simulink model "i_r303_med_1"  (Simulink 6.2)
settings: Solver=ode45  StartTime=0.0  StopTime=10  RelTol=1e-3
libraries: xbsIndex_r3 x540, xps_library x26, ddc_library x4, reorder_library x3, fft_library x2, pfb_library x2, simulink x1, adcscope_lib x1, delay_lib x1
(part 1 of 4)
settings Model: LastModifiedBy=dsp
settings DebuggingCC: SolverPrmCheckMsg=warning

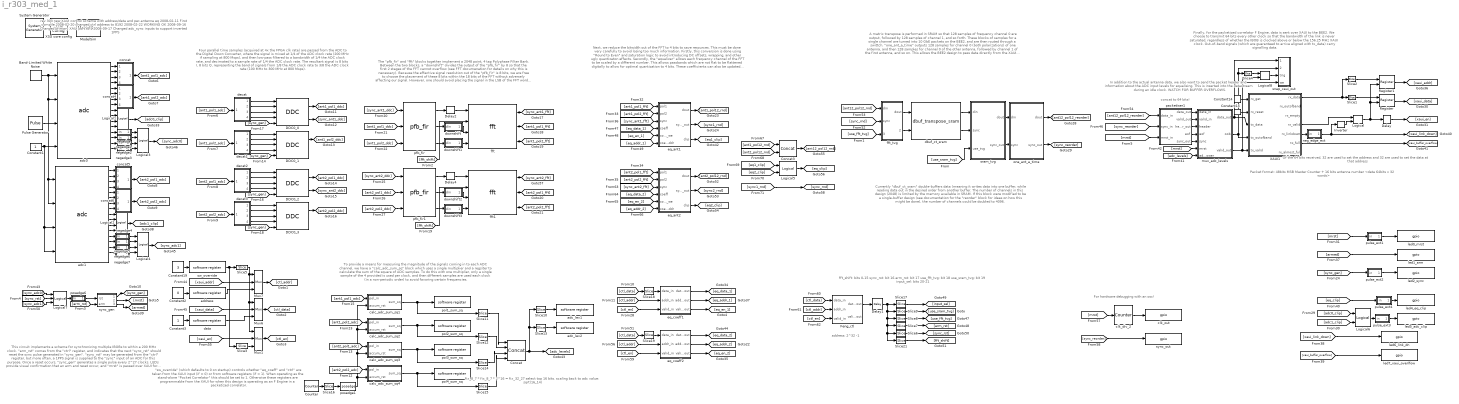
== system i_r303_med_1 ==
  note: rev 303
      | new XAUI control scheme with address/data
      | and per-antenna eq
      | 2008-02-11 First compile
      | 2008-02-20 changed ctrl address to 8192
      | 2008-02-22 WORKING OK
      | 2008-09-16 Changed primary XAUI port to 1
      | 2008-09-17 Changed adc_sync inputs to support inverted 1PPS
  note: This circuit implements a scheme for synchronizing
      | multiple IBOBs to within a 200 MHz clock.  "arm_rst"
      | comes from the "ctrl" register, and indicates that the
      | next "sync_rst" should reset the sync pulse generated
      | in "sync_gen".  "sync_rst" may be generated from
      | the "ctrl" register, but more often, a 1PPS signal is
      | supplied to the "sync" input of an ADC for this
      | purpose.  Once a reset occurs, "sync_gen" generates
      | a single pulse every 2^27 clocks.  LEDs provide visual
      | confirmation that an arm and reset occur, and "mrst"
      | is passed over XAUI for the purpose of informing
      | downstream logic in a packetized correlator that
      | a "master reset" has occurred.
  note: "sw_override" (which defaults to 0 on startup)
      | controls whether "eq_coeff" and "ctrl" are taken
      | from the XAUI input (if = 0) or from software
      | registers (if = 1).  When operating as the stand-alone
      | "Pocket Correlator" this should be set to 1.  Otherwise
      | these registers are programmable from the XAUI for
      | when this design is operating as  an F Engine
      | in a packetized correlator.
  note: Four parallel time samples (acquired at 4x the
      | FPGA clk rate) are passed from the ADC to the
      | Digital Down Converter, where the signal is mixed
      | at 1/4 of the ADC clock rate (200 MHz if sampling
      | at 800 Msps), and then low-pass filtered to a
      | bandwidth of 1/4 the ADC clock rate, and decimated
      | to a sample rate of 1/4 the ADC clock rate.  The
      | resultant signal is 8 bits I, 8 bits Q, representing the
      | band of signals from 1/8 the ADC clock rate to
      | 3/8 the ADC clock rate (100 MHz to 300 MHz at
      | 800 Msps).
  note: The "pfb_fir" and "fft" blocks together implement a 2048 point,
      | 4 tap Polyphase Filter Bank.  Between the two blocks, a "downshift"
      | divides the output of the "pfb_fir" by 8 so that the first 2 stages of
      | the FFT cannot overflow (see FFT documenation for details on why
      | this is necessary).  Because the effective signal resolution out of
      | the "pfb_fir" is 8 bits, we are free to choose the placement of
      | these 8 bits within the 18 bits of the FFT without adversely affecting
      | our signal.  However, one should avoid placing the signal in the LSB
      | of the FFT word because of rounding effects.  Thus, we downshift
      | only 3 bits.
  note: Next, we reduce the bitwidth out of the FFT to 4 bits to save resources.
      | This must be done very carefully to avoid losing too much information.
      | Firstly, this conversion is done using "Round to Even" and saturation
      | logic to avoid introducing DC offsets, wrapping, and other ugly quantizaton
      | effects.  Secondly, the "equalizer" allows each frequency channel of the
      | FFT to be scaled by a different number.  This allows passbands which are
      | not flat to be flattened digitally to allow for optimal quantization to 4 bits.
      | These coefficients can also be updated dynamically for gain control.
      | Coefficients can be dynamically written into the "equalizer" by
      | specifying the channel ("coeff_addr") and the value of the
      | coefficient ("coeff"), and then using "coeff_en" to write the
      | new coefficient into the equalization table.
  note: To provide a means for measuring the magnitude of the signals
      | coming in to each ADC channel, we have a "calc_adc_sum_sq"
      | block which uses a single multiplier and a regsiter to calculate
      | the sum of the square of ADC samples.  To do this with one
      | multiplier, only a single sample of the 4 provided is used
      | per clock, and then different samples are used each clock (in
      | a non-periodic order) to avoid favoring certain frequencies.
  note: A matrix transpose is performed in SRAM so that 128 samples of frequency
      | channel 0 are output, followed by 128 samples of channel 1, and so forth.
      | These blocks of samples for a single channel are turned into 10 GbE packets
      | on the BEE2, and are then routed through a swittch.  "one_ant_a_time"
      | outputs 128 samples for channel 0 (both polarizations) of one antenna,
      | and then 128 samples for channel 0 of the other antenna, followed by
      | channel 1 of the first antenna, and so on.  This allows the BEE2 design to
      | pass data directly from the XAUI into a packet containing 128 time samples
      | for 1 frequency from 1 antenna.
  note: Currently "dbuf_ct_sram" double-buffers data (meaning it writes data
      | into one buffer, while reading data out in the desired order from another
      | buffer.  The number of channels in this design (2048) is limited by the
      | memory available in SRAM.  If this block were modified to be a
      | single-buffer design (see documentation for the "reorder" block for
      | ideas on how this might be done), the number of channels could
      | be doubled to 4096.
  note: Finally, for the packetized correlator F Engine, data is sent over
      | XAUI to the BEE2.  We choose to transmit 64 bits every other clock
      | so that the bandwidth of the link is never saturated, regardless of whether
      | the IBOB is clocked above or below the 156.25 MHz XAUI clock.
      | Out-of-band signals (which are guaranteed to arrive aligned with
      | tx_data) carry signalling data.
  note: Of the 64 bits received, 32 are used to set the address
      | and 32 are used to set the data at that address
  note: fix_8_7 * fix_8_7 * 2^16 = fix_32_27
      | select top 16 bits.
      | scaling back to adc value: sqrt(16_14)
  note: In addition to the actual antenna data,
      | we also want to send the packet header
      | and information about the ADC input levels for equalising.
      | This is inserted into the datastream during an idle clock.
      | WATCH FOR BUFFER OVERFLOWS.
  note: Packet format:
      | 48bits MSB Master Counter + 16 bits antenna number
      | <data 64bits x 32 words>
  note: concat to 64 bits!
  note: fft_shift: bits 0-15
      | sync_rst: bit 16
      | arm_rst: bit 17
      | use_fft_tvg: bit 18
      | use_sram_tvg: bit 19
      | input_sel: bits 20-21
  note: For hardware debugging with an osc!
  note: address: 2^32 -1
  " System Generator" : xbsIndex_r3/ System Generator  Tag=genX  xilinxfamily=Virtex2P  part=xc2vp50  speed=-7  package=ff1152  synthesis_tool=XST  directory=./i_r303_med_1/sysgen  testbench=off  simulink_period=1  sysclk_period=5  incr_netlist=off  trim_vbits=Everywhere in SubSystem  dbl_ovrd=According to Block Masks  core_generation=According to Block Masks  run_coregen=off  deprecated_control=off  eval_field=0
      settings: AttributesFormatString=System\nGenerator
  Band-Limited White Noise : simulink/Sources/Band-Limited White Noise  Cov=[0.1]  Ts=0.1  seed=[23341]
  Concat : xbsIndex_r3/Concat  num_inputs=4  explicit_period=off  period=1  dbl_ovrd=off
  Concat3 : xbsIndex_r3/Concat  num_inputs=2  explicit_period=off  period=1  dbl_ovrd=off
  Constant1 : Constant
  Constant14 : xbsIndex_r3/Constant  const=1  equ=P=C  arith_type=Unsigned  n_bits=1  bin_pt=0  opselect=C  inp2=PCIN>>17  opr=+  inp1=P  carry=CIN  iostate=0  explicit_period=on  period=1  dbl_ovrd=off
  Constant15 : xbsIndex_r3/Constant  const=0  equ=P=C  arith_type=Unsigned  n_bits=1  bin_pt=0  opselect=C  inp2=PCIN>>17  opr=+  inp1=P  carry=CIN  iostate=0  explicit_period=on  period=1  dbl_ovrd=off
  Constant19 : Constant  Value=3
  Constant2 : Constant  Value=0
  Constant3 : Constant
  Counter : xbsIndex_r3/Counter  cnt_type=Free Running  n_bits=16  bin_pt=0  arith_type=Unsigned  start_count=0  cnt_to=Inf  cnt_by_val=1  operation=Up  explicit_period=off  period=1  load_pin=off  rst=off  en=off  dbl_ovrd=off  show_param=off  use_rpm=on  gen_core=off
      settings: xl_area=[0, 0, 0, 0, 0, 0, 0]
  DDC0_{0..3} (4 alike) : ddc_library/DDC  freq_div=4  lo_freq=1  num_inputs=4  lo_bitwidth=8  lpfir_coeff=".9 * [-0.0161   -0.0428   -0.0504   -0.0249    0.0354    0.1170    0.1948    0.2422    0.2422    0.1948    0.1170  0.0354   -0.0249   -0.0504   -0.0428   -0.0161]"  BitWidthOut=8  quantization="Round  (unbiased: Even Values)"  add_latency=1  mult_latency=2
  Delay : xbsIndex_r3/Delay  latency=1  reg_retiming=off  explicit_period=off  period=1  en=off  accept_only_valid=off  init_zero=on  dbl_ovrd=off  show_param=off
      settings: xl_area=[0, 0, 0, 0, 0, 0, 0]
  Delay1 : xbsIndex_r3/Delay  latency=1  reg_retiming=off  explicit_period=off  period=1  en=off  accept_only_valid=off  init_zero=on  dbl_ovrd=off  show_param=off
      settings: xl_area=[0, 0, 0, 0, 0, 0, 0]
  Delay2 : xbsIndex_r3/Delay  latency=2  reg_retiming=off  explicit_period=off  period=1  en=off  accept_only_valid=off  init_zero=on  dbl_ovrd=off  show_param=off
      settings: xl_area=[0, 0, 0, 0, 0, 0, 0]
  Delay4 : xbsIndex_r3/Delay  latency=2  reg_retiming=off  explicit_period=off  period=1  en=off  accept_only_valid=off  init_zero=on  dbl_ovrd=off  show_param=off
      settings: xl_area=[0, 0, 0, 0, 0, 0, 0]
  Feng_ctl : Subsystem  mask{addr_offset=8192}
      mask prompts: addr_offset "Address"
      mask init:
      | start_addr = (addr_offset);
      | fmtstr = sprintf('Mapped address: %d', start_addr);
      | set_param(gcb, 'AttributesFormatString', fmtstr);
      settings: AttributesFormatString=Mapped address: 8192
  Inverter : xbsIndex_r3/Inverter  latency=0  explicit_period=off  period=1  en=off  dbl_ovrd=off  show_param=off
      settings: xl_area=[0, 0, 0, 0, 0, 0, 0]
  Logical : xbsIndex_r3/Logical  logical_function=AND  inputs=2  precision=Full  arith_type=Unsigned  n_bits=8  bin_pt=2  align_bp=on  latency=0  explicit_period=off  period=1  en=off  dbl_ovrd=off  show_param=off
      settings: xl_area=[0, 0, 0, 0, 0, 0, 0]
  Logical{1..4} (4 alike) : xbsIndex_r3/Logical  logical_function=OR  inputs=4  precision=Full  arith_type=Unsigned  n_bits=8  bin_pt=2  align_bp=on  latency=1  explicit_period=off  period=1  en=off  dbl_ovrd=off  show_param=off
      settings: xl_area=[0, 0, 0, 0, 0, 0, 0]
  Logical5 : xbsIndex_r3/Logical  logical_function=OR  inputs=2  precision=Full  arith_type=Unsigned  n_bits=8  bin_pt=2  align_bp=on  latency=0  explicit_period=off  period=1  en=off  dbl_ovrd=off  show_param=off
      settings: xl_area=[0, 0, 0, 0, 0, 0, 0]
  Logical6 : xbsIndex_r3/Logical  logical_function=OR  inputs=2  precision=Full  arith_type=Unsigned  n_bits=8  bin_pt=2  align_bp=on  latency=1  explicit_period=off  period=1  en=off  dbl_ovrd=off  show_param=off
      settings: xl_area=[0, 0, 0, 0, 0, 0, 0]
  Logical7 : xbsIndex_r3/Logical  logical_function=OR  inputs=3  precision=Full  arith_type=Unsigned  n_bits=8  bin_pt=2  align_bp=on  latency=1  explicit_period=off  period=1  en=off  dbl_ovrd=off  show_param=off
      settings: xl_area=[0, 0, 0, 0, 0, 0, 0]
  Logical8 : xbsIndex_r3/Logical  logical_function=AND  inputs=2  precision=Full  arith_type=Unsigned  n_bits=8  bin_pt=2  align_bp=on  latency=0  explicit_period=off  period=1  en=off  dbl_ovrd=off  show_param=off
      settings: xl_area=[0, 0, 0, 0, 0, 0, 0]
  ModelSim : xbsIndex_r3/ModelSim  dir=./modelsim  waveform=on  leave_open=on  skip_compile=off  custom_scripts=off  startup_timeout=40
  Mux1 : xbsIndex_r3/Mux  inputs=2  precision=Full  arith_type="Signed  (2's comp)"  n_bits=8  bin_pt=2  quantization=Truncate  overflow=Wrap  latency=1  explicit_period=on  period=1  en=off  dbl_ovrd=off  show_param=off  mux_type=off  use_rpm=off  gen_core=off
      settings: xl_area=[0, 0, 0, 0, 0, 0, 0]
  Mux6 : xbsIndex_r3/Mux  inputs=2  precision=Full  arith_type="Signed  (2's comp)"  n_bits=8  bin_pt=2  quantization=Truncate  overflow=Wrap  latency=1  explicit_period=on  period=1  en=off  dbl_ovrd=off  show_param=off  mux_type=off  use_rpm=off  gen_core=off
      settings: xl_area=[0, 0, 0, 0, 0, 0, 0]
  Mux7 : xbsIndex_r3/Mux  inputs=2  precision=Full  arith_type="Signed  (2's comp)"  n_bits=8  bin_pt=2  quantization=Truncate  overflow=Wrap  latency=1  explicit_period=on  period=1  en=off  dbl_ovrd=off  show_param=off  mux_type=off  use_rpm=off  gen_core=off
      settings: xl_area=[0, 0, 0, 0, 0, 0, 0]
  Pulse Generator : DiscretePulseGenerator  Period=2^27
  Register : xbsIndex_r3/Register  init=0  reg_only_valid=off  explicit_period=off  period=1  rst=off  en=on  out_en=off  dbl_ovrd=off  show_param=off
      settings: xl_area=[0, 0, 0, 0, 0, 0, 0]
  Register1 : xbsIndex_r3/Register  init=0  reg_only_valid=off  explicit_period=off  period=1  rst=off  en=on  out_en=off  dbl_ovrd=off  show_param=off
      settings: xl_area=[0, 0, 0, 0, 0, 0, 0]
  Slice1 : xbsIndex_r3/Slice  mode=Lower Bit Location + Width  nbits=32  bit1=0  base1=MSB of Input  bit0=0  base0=LSB of Input  boolean_output=on  explicit_period=off  period=1  dbl_ovrd=off
  Slice10 : xbsIndex_r3/Slice  mode=Lower Bit Location + Width  nbits=32  bit1=0  base1=MSB of Input  bit0=0  base0=LSB of Input  boolean_output=off  explicit_period=off  period=1  dbl_ovrd=off
  Slice{11..12,14..15} (4 alike) : xbsIndex_r3/Slice  mode=Upper Bit Location + Width  nbits=16  bit1=0  base1=MSB of Input  bit0=0  base0=LSB of Input  boolean_output=off  explicit_period=off  period=1  dbl_ovrd=off
  Slice13 : xbsIndex_r3/Slice  mode=Lower Bit Location + Width  nbits=32  bit1=0  base1=MSB of Input  bit0=32  base0=LSB of Input  boolean_output=off  explicit_period=off  period=1  dbl_ovrd=off
  Slice16 : xbsIndex_r3/Slice  mode=Upper Bit Location + Width  nbits=1  bit1=0  base1=MSB of Input  bit0=19  base0=LSB of Input  boolean_output=on  explicit_period=off  period=1  dbl_ovrd=off
  Slice17 : xbsIndex_r3/Slice  mode=Lower Bit Location + Width  nbits=2  bit1=0  base1=MSB of Input  bit0=20  base0=LSB of Input  boolean_output=off  explicit_period=off  period=1  dbl_ovrd=off
  Slice18 : xbsIndex_r3/Slice  mode=Lower Bit Location + Width  nbits=17  bit1=0  base1=MSB of Input  bit0=0  base0=LSB of Input  boolean_output=off  explicit_period=off  period=1  dbl_ovrd=off
  Slice19 : xbsIndex_r3/Slice  mode=Lower Bit Location + Width  nbits=17  bit1=0  base1=MSB of Input  bit0=0  base0=LSB of Input  boolean_output=off  explicit_period=off  period=1  dbl_ovrd=off
  Slice2 : xbsIndex_r3/Slice  mode=Lower Bit Location + Width  nbits=32  bit1=0  base1=MSB of Input  bit0=32  base0=LSB of Input  boolean_output=off  explicit_period=off  period=1  dbl_ovrd=off
  Slice21 : xbsIndex_r3/Slice  mode=Lower Bit Location + Width  nbits=16  bit1=0  base1=MSB of Input  bit0=0  base0=LSB of Input  boolean_output=off  explicit_period=off  period=1  dbl_ovrd=off
  Slice3 : xbsIndex_r3/Slice  mode=Lower Bit Location + Width  nbits=1  bit1=0  base1=MSB of Input  bit0=1  base0=LSB of Input  boolean_output=on  explicit_period=off  period=1  dbl_ovrd=off
  Slice4 : xbsIndex_r3/Slice  mode=Lower Bit Location + Width  nbits=1  bit1=0  base1=MSB of Input  bit0=1  base0=LSB of Input  boolean_output=on  explicit_period=off  period=1  dbl_ovrd=off
  Slice5 : xbsIndex_r3/Slice  mode=Lower Bit Location + Width  nbits=1  bit1=0  base1=MSB of Input  bit0=0  base0=LSB of Input  boolean_output=off  explicit_period=off  period=1  dbl_ovrd=off
  Slice6 : xbsIndex_r3/Slice  mode=Lower Bit Location + Width  nbits=1  bit1=0  base1=MSB of Input  bit0=16  base0=LSB of Input  boolean_output=on  explicit_period=off  period=1  dbl_ovrd=off
  Slice7 : xbsIndex_r3/Slice  mode=Lower Bit Location + Width  nbits=1  bit1=0  base1=MSB of Input  bit0=17  base0=LSB of Input  boolean_output=on  explicit_period=off  period=1  dbl_ovrd=off
  Slice8 : xbsIndex_r3/Slice  mode=Lower Bit Location + Width  nbits=1  bit1=0  base1=MSB of Input  bit0=18  base0=LSB of Input  boolean_output=off  explicit_period=off  period=1  dbl_ovrd=off
  Slice9 : xbsIndex_r3/Slice  mode=Lower Bit Location + Width  nbits=1  bit1=0  base1=MSB of Input  bit0=19  base0=LSB of Input  boolean_output=off  explicit_period=off  period=1  dbl_ovrd=off
  XAUI1 : Subsystem  Tag=xps:xaui  AncestorBlock=xps_library/XAUI  mask{demux=1, port=iBOB:1, show_param=off, pre_emph=3, swing=800}
      mask prompts: show_param "---------------------- Show Implementation Parameters -----------------------------------------------------------------------------------"; pre_emph "Pre-emphasis"; swing "Differential swing"
      mask init:
      | xaui_mask;
      mask StyleString: popup(1|2),popup(iBOB:0|iBOB:1|BEE2_ctrl:0|BEE2_ctrl:1|BEE2_usr:0|BEE2_usr:1|BEE2_usr:2|BEE2_usr:3|CORR:0),checkbox,popup(0|1|2|3),popup(400|500|600|700|800)
      mask CallbackString:
      | ||myname=gcb;
      | if strcmp(get_param(myname, 'show_param'), 'on')
      |     set_param(myname, 'MaskVisibilities', {'on','on','on','on','on'});
      | else
      |     set_param(myname, 'MaskVisibilities', {'on','on','on','off','off'});
      | end||
  XSG core config : xps_library/XSG core config  Tag=xps:xsg  hw_sys=iBOB  ibob_linux=off  clk_src=adc0_clk  gpio_clk_io_group=iBOB:sma  gpio_clk_bit_index=0  clk_rate=200  sample_period=1  synthesis_tool=XST  mpc_type=powerpc405
  adc0 : xps_library/adc  Tag=xps:adc  adc_brd=iBOB:adc0  adc_clk_rate=600  adc_interleave=off  sample_period=1
  adc1 : xps_library/adc  Tag=xps:adc  adc_brd=iBOB:adc1  adc_clk_rate=600  adc_interleave=off  sample_period=1
  adc_lev1 : xps_library/software register  Tag=xps:sw_reg  io_dir=To Processor  arith_type=Unsigned  bitwidth=32  bin_pt=14  sample_period=1  gw_name=i_r303_med_1_adc_lev1_user_data_in
  adc_lev2 : xps_library/software register  Tag=xps:sw_reg  io_dir=To Processor  arith_type=Unsigned  bitwidth=32  bin_pt=14  sample_period=1  gw_name=i_r303_med_1_adc_lev2_user_data_in
  address : xps_library/software register  Tag=xps:sw_reg  io_dir=From Processor  arith_type=Unsigned  bitwidth=32  bin_pt=0  sample_period=1  gw_name=i_r303_med_1_address_user_data_out
  calc_adc_sum_sq1 : Subsystem
  calc_adc_sum_sq2 : Subsystem
  calc_adc_sum_sq3 : Subsystem
  calc_adc_sum_sq4 : Subsystem
  clk_div_2 : xbsIndex_r3/Counter  cnt_type=Free Running  n_bits=1  bin_pt=0  arith_type=Unsigned  start_count=0  cnt_to=Inf  cnt_by_val=1  operation=Up  explicit_period=off  period=1  load_pin=off  rst=on  en=off  dbl_ovrd=off  show_param=off  use_rpm=on  gen_core=off
      settings: xl_area=[0, 0, 0, 0, 0, 0, 0]
  clk_out : xps_library/gpio  Tag=xps:gpio  io_group=iBOB:sma  io_dir=out  arith_type=Unsigned  bitwidth=1  bin_pt=0  bit_index=0  sample_period=1  use_single_ended=off  use_ddr=off  reg_iob=on  reg_clk_phase=0  termination=None
  concat : Subsystem
  concat4 : Subsystem
  concat5 : Subsystem
  concat6 : Subsystem
  data : xps_library/software register  Tag=xps:sw_reg  io_dir=From Processor  arith_type=Unsigned  bitwidth=32  bin_pt=0  sample_period=1  gw_name=i_r303_med_1_data_user_data_out
  dbuf_ct_sram : reorder_library/dbuf_transpose_sram  length=2^11  numSpecs=128
      link override sync_delay/Constant: equ=P=C
      link override sync_delay/Constant1: equ=P=C
      link override sync_delay/Constant2: equ=P=C
      link override sync_delay/Constant3: equ=P=C
  decat : Subsystem
  decat1 : Subsystem
  decat2 : Subsystem
  decat3 : Subsystem
  downshift : Subsystem
  downshift1 : Subsystem
  downshift2 : Subsystem
  downshift3 : Subsystem
  eq_ant1 : Subsystem
  eq_ant2 : Subsystem
  eq_coeff1 : Subsystem  mask{addr_width=11, addr_offset=0}
      mask prompts: addr_width "Number of addresses (2^?)"; addr_offset "Address block offset (multiple of above)"
      mask init:
      | start_addr = 2^addr_width*(addr_offset);
      | end_addr = start_addr + 2^addr_width - 1;
      | fmtstr = sprintf('Mapped address range: %d-%d', start_addr,end_addr);
      | set_param(gcb, 'AttributesFormatString', fmtstr);
      settings: AttributesFormatString=Mapped address range: 0-2047
  eq_coeff2 : Subsystem  mask{addr_width=11, addr_offset=1}
      mask prompts: addr_width "Number of addresses (2^?)"; addr_offset "Address block offset (multiple of above)"
      mask init: same as i_r303_med_1/eq_coeff1
      settings: AttributesFormatString=Mapped address range: 2048-4095
  fft : fft_library/fft  FFTSize=11  BitWidth=18  n_inputs=0  quantization="Round  (unbiased: Even Values)"  overflow=Wrap  add_latency=1  mult_latency=2  bram_latency=2
  fft1 : fft_library/fft  FFTSize=11  BitWidth=18  n_inputs=0  quantization="Round  (unbiased: Even Values)"  overflow=Wrap  add_latency=1  mult_latency=2  bram_latency=2
  fft_tvg : Subsystem
  led0_mrst : xps_library/gpio  Tag=xps:gpio  io_group=iBOB:led  io_dir=out  arith_type=Boolean  bitwidth=1  bin_pt=0  bit_index=0  sample_period=1  use_single_ended=off  use_ddr=off  reg_iob=on  reg_clk_phase=0  termination=None
  led1_arm : xps_library/gpio  Tag=xps:gpio  io_group=iBOB:led  io_dir=out  arith_type=Boolean  bitwidth=1  bin_pt=0  bit_index=1  sample_period=1  use_single_ended=off  use_ddr=off  reg_iob=on  reg_clk_phase=0  termination=None
  led2_sync : xps_library/gpio  Tag=xps:gpio  io_group=iBOB:led  io_dir=out  arith_type=Boolean  bitwidth=1  bin_pt=0  bit_index=2  sample_period=1  use_single_ended=off  use_ddr=off  reg_iob=on  reg_clk_phase=0  termination=None
  led4_eq_clip : xps_library/gpio  Tag=xps:gpio  io_group=iBOB:led  io_dir=out  arith_type=Boolean  bitwidth=1  bin_pt=0  bit_index=4  sample_period=1  use_single_ended=off  use_ddr=off  reg_iob=on  reg_clk_phase=0  termination=None
  led5_adc_clip : xps_library/gpio  Tag=xps:gpio  io_group=iBOB:led  io_dir=out  arith_type=Boolean  bitwidth=1  bin_pt=0  bit_index=5  sample_period=1  use_single_ended=off  use_ddr=off  reg_iob=on  reg_clk_phase=0  termination=None
  led6_link_dn : xps_library/gpio  Tag=xps:gpio  io_group=iBOB:led  io_dir=out  arith_type=Unsigned  bitwidth=1  bin_pt=0  bit_index=6  sample_period=1  use_single_ended=off  use_ddr=off  reg_iob=on  reg_clk_phase=0  termination=None
  led7_xaui_overlfow : xps_library/gpio  Tag=xps:gpio  io_group=iBOB:led  io_dir=out  arith_type=Unsigned  bitwidth=1  bin_pt=0  bit_index=7  sample_period=1  use_single_ended=off  use_ddr=off  reg_iob=on  reg_clk_phase=0  termination=None
  mux_adc_levels : Subsystem  mask{wait_time=2000}
      mask prompts: wait_time "Attempt to insert antenna levels how many clocks after sync?"
  neg_edge_ext : Subsystem  mask{pulse_len=2^27}
      mask prompts: pulse_len "Length of Pulse"
      mask init:
      | bits = ceil(log2(pulse_len+1));
  negedge : Subsystem  Tag=Rising Edge Detector
  negedge1 : Subsystem  Tag=Rising Edge Detector
  negedge2 : Subsystem  Tag=Rising Edge Detector
  negedge3 : Subsystem  Tag=Rising Edge Detector
  negedge4 : Subsystem  Tag=Rising Edge Detector
  negedge5 : Subsystem  Tag=Rising Edge Detector
  negedge6 : Subsystem  Tag=Rising Edge Detector
  negedge7 : Subsystem  Tag=Rising Edge Detector
  one_ant_a_time : Subsystem
  packetiser1 : Subsystem  mask{nwrd_bits=5, ant_bits=1}
      mask prompts: nwrd_bits "Payload length: (in 64bit words) (2^n)"; ant_bits "Number of antennas on this link (2^n)"
      mask help: Package 32 bit data into 64 bits and identify data as coming from antenna 0 or 1
  pfb_fir : pfb_library/pfb_fir  PFBSize=11  TotalTaps=4  WindowType=hamming  n_inputs=0  MakeBiplex=on  BitWidthIn=8  BitWidthOut=18  CoeffBitWidth=8  CoeffDistMem=off  add_latency=1  mult_latency=2  bram_latency=2  quantization="Round  (unbiased: Even Values)"  fwidth=1
      link override pol1_in1_first_tap/sync_delay/Constant: equ=P=C
      link override pol1_in1_first_tap/sync_delay/Constant1: equ=P=C
      link override pol1_in1_first_tap/sync_delay/Constant2: equ=P=C
      link override pol1_in1_first_tap/sync_delay/Constant3: equ=P=C
      link override pol1_in1_tap10/sync_delay/Constant: equ=P=C
      link override pol1_in1_tap10/sync_delay/Constant1: equ=P=C
      link override pol1_in1_tap10/sync_delay/Constant2: equ=P=C
      link override pol1_in1_tap10/sync_delay/Constant3: equ=P=C
      link override pol1_in1_tap11/sync_delay/Constant: equ=P=C
      link override pol1_in1_tap11/sync_delay/Constant1: equ=P=C
      link override pol1_in1_tap11/sync_delay/Constant2: equ=P=C
      link override pol1_in1_tap11/sync_delay/Constant3: equ=P=C
      link override pol1_in1_tap12/sync_delay/Constant: equ=P=C
      link override pol1_in1_tap12/sync_delay/Constant1: equ=P=C
      link override pol1_in1_tap12/sync_delay/Constant2: equ=P=C
      link override pol1_in1_tap12/sync_delay/Constant3: equ=P=C
      link override pol1_in1_tap13/sync_delay/Constant: equ=P=C
      link override pol1_in1_tap13/sync_delay/Constant1: equ=P=C
      link override pol1_in1_tap13/sync_delay/Constant2: equ=P=C
      link override pol1_in1_tap13/sync_delay/Constant3: equ=P=C
      link override pol1_in1_tap14/sync_delay/Constant: equ=P=C
      link override pol1_in1_tap14/sync_delay/Constant1: equ=P=C
      link override pol1_in1_tap14/sync_delay/Constant2: equ=P=C
      link override pol1_in1_tap14/sync_delay/Constant3: equ=P=C
      link override pol1_in1_tap15/sync_delay/Constant: equ=P=C
      link override pol1_in1_tap15/sync_delay/Constant1: equ=P=C
      link override pol1_in1_tap15/sync_delay/Constant2: equ=P=C
      link override pol1_in1_tap15/sync_delay/Constant3: equ=P=C
      link override pol1_in1_tap2/sync_delay/Constant: equ=P=C
      link override pol1_in1_tap2/sync_delay/Constant1: equ=P=C
      link override pol1_in1_tap2/sync_delay/Constant2: equ=P=C
      link override pol1_in1_tap2/sync_delay/Constant3: equ=P=C
      link override pol1_in1_tap3/sync_delay/Constant: equ=P=C
      link override pol1_in1_tap3/sync_delay/Constant1: equ=P=C
      link override pol1_in1_tap3/sync_delay/Constant2: equ=P=C
      link override pol1_in1_tap3/sync_delay/Constant3: equ=P=C
      link override pol1_in1_tap4/sync_delay/Constant: equ=P=C
      link override pol1_in1_tap4/sync_delay/Constant1: equ=P=C
      link override pol1_in1_tap4/sync_delay/Constant2: equ=P=C
      link override pol1_in1_tap4/sync_delay/Constant3: equ=P=C
      link override pol1_in1_tap5/sync_delay/Constant: equ=P=C
      link override pol1_in1_tap5/sync_delay/Constant1: equ=P=C
      link override pol1_in1_tap5/sync_delay/Constant2: equ=P=C
      link override pol1_in1_tap5/sync_delay/Constant3: equ=P=C
      link override pol1_in1_tap6/sync_delay/Constant: equ=P=C
      link override pol1_in1_tap6/sync_delay/Constant1: equ=P=C
      link override pol1_in1_tap6/sync_delay/Constant2: equ=P=C
      link override pol1_in1_tap6/sync_delay/Constant3: equ=P=C
      link override pol1_in1_tap7/sync_delay/Constant: equ=P=C
      link override pol1_in1_tap7/sync_delay/Constant1: equ=P=C
      link override pol1_in1_tap7/sync_delay/Constant2: equ=P=C
      link override pol1_in1_tap7/sync_delay/Constant3: equ=P=C
      link override pol1_in1_tap8/sync_delay/Constant: equ=P=C
      link override pol1_in1_tap8/sync_delay/Constant1: equ=P=C
      link override pol1_in1_tap8/sync_delay/Constant2: equ=P=C
      link override pol1_in1_tap8/sync_delay/Constant3: equ=P=C
      link override pol1_in1_tap9/sync_delay/Constant: equ=P=C
      link override pol1_in1_tap9/sync_delay/Constant1: equ=P=C
      link override pol1_in1_tap9/sync_delay/Constant2: equ=P=C
      link override pol1_in1_tap9/sync_delay/Constant3: equ=P=C
      link override pol2_in1_first_tap/sync_delay/Constant: equ=P=C
      link override pol2_in1_first_tap/sync_delay/Constant1: equ=P=C
      link override pol2_in1_first_tap/sync_delay/Constant2: equ=P=C
      link override pol2_in1_first_tap/sync_delay/Constant3: equ=P=C
      link override pol2_in1_tap10/sync_delay/Constant: equ=P=C
      link override pol2_in1_tap10/sync_delay/Constant1: equ=P=C
      link override pol2_in1_tap10/sync_delay/Constant2: equ=P=C
      link override pol2_in1_tap10/sync_delay/Constant3: equ=P=C
      link override pol2_in1_tap11/sync_delay/Constant: equ=P=C
      link override pol2_in1_tap11/sync_delay/Constant1: equ=P=C
      link override pol2_in1_tap11/sync_delay/Constant2: equ=P=C
      link override pol2_in1_tap11/sync_delay/Constant3: equ=P=C
      link override pol2_in1_tap12/sync_delay/Constant: equ=P=C
      link override pol2_in1_tap12/sync_delay/Constant1: equ=P=C
      link override pol2_in1_tap12/sync_delay/Constant2: equ=P=C
      link override pol2_in1_tap12/sync_delay/Constant3: equ=P=C
      link override pol2_in1_tap13/sync_delay/Constant: equ=P=C
      link override pol2_in1_tap13/sync_delay/Constant1: equ=P=C
      link override pol2_in1_tap13/sync_delay/Constant2: equ=P=C
      link override pol2_in1_tap13/sync_delay/Constant3: equ=P=C
      link override pol2_in1_tap14/sync_delay/Constant: equ=P=C
      link override pol2_in1_tap14/sync_delay/Constant1: equ=P=C
      link override pol2_in1_tap14/sync_delay/Constant2: equ=P=C
      link override pol2_in1_tap14/sync_delay/Constant3: equ=P=C
      link override pol2_in1_tap15/sync_delay/Constant: equ=P=C
      link override pol2_in1_tap15/sync_delay/Constant1: equ=P=C
      link override pol2_in1_tap15/sync_delay/Constant2: equ=P=C
      link override pol2_in1_tap15/sync_delay/Constant3: equ=P=C
      link override pol2_in1_tap2/sync_delay/Constant: equ=P=C
      link override pol2_in1_tap2/sync_delay/Constant1: equ=P=C
      link override pol2_in1_tap2/sync_delay/Constant2: equ=P=C
      link override pol2_in1_tap2/sync_delay/Constant3: equ=P=C
      link override pol2_in1_tap3/sync_delay/Constant: equ=P=C
      link override pol2_in1_tap3/sync_delay/Constant1: equ=P=C
      link override pol2_in1_tap3/sync_delay/Constant2: equ=P=C
      link override pol2_in1_tap3/sync_delay/Constant3: equ=P=C
      link override pol2_in1_tap4/sync_delay/Constant: equ=P=C
      link override pol2_in1_tap4/sync_delay/Constant1: equ=P=C
      link override pol2_in1_tap4/sync_delay/Constant2: equ=P=C
      link override pol2_in1_tap4/sync_delay/Constant3: equ=P=C
      link override pol2_in1_tap5/sync_delay/Constant: equ=P=C
      link override pol2_in1_tap5/sync_delay/Constant1: equ=P=C
      link override pol2_in1_tap5/sync_delay/Constant2: equ=P=C
      link override pol2_in1_tap5/sync_delay/Constant3: equ=P=C
      link override pol2_in1_tap6/sync_delay/Constant: equ=P=C
      link override pol2_in1_tap6/sync_delay/Constant1: equ=P=C
      link override pol2_in1_tap6/sync_delay/Constant2: equ=P=C
      link override pol2_in1_tap6/sync_delay/Constant3: equ=P=C
      link override pol2_in1_tap7/sync_delay/Constant: equ=P=C
      link override pol2_in1_tap7/sync_delay/Constant1: equ=P=C
      link override pol2_in1_tap7/sync_delay/Constant2: equ=P=C
      link override pol2_in1_tap7/sync_delay/Constant3: equ=P=C
      link override pol2_in1_tap8/sync_delay/Constant: equ=P=C
      link override pol2_in1_tap8/sync_delay/Constant1: equ=P=C
      link override pol2_in1_tap8/sync_delay/Constant2: equ=P=C
      link override pol2_in1_tap8/sync_delay/Constant3: equ=P=C
      link override pol2_in1_tap9/sync_delay/Constant: equ=P=C
      link override pol2_in1_tap9/sync_delay/Constant1: equ=P=C
      link override pol2_in1_tap9/sync_delay/Constant2: equ=P=C
      link override pol2_in1_tap9/sync_delay/Constant3: equ=P=C
  pfb_fir1 : pfb_library/pfb_fir  PFBSize=11  TotalTaps=4  WindowType=hamming  n_inputs=0  MakeBiplex=on  BitWidthIn=8  BitWidthOut=18  CoeffBitWidth=8  CoeffDistMem=off  add_latency=1  mult_latency=2  bram_latency=2  quantization="Round  (unbiased: Even Values)"  fwidth=1
      link override pol1_in1_first_tap/sync_delay/Constant: equ=P=C
      link override pol1_in1_first_tap/sync_delay/Constant1: equ=P=C
      link override pol1_in1_first_tap/sync_delay/Constant2: equ=P=C
      link override pol1_in1_first_tap/sync_delay/Constant3: equ=P=C
      link override pol1_in1_tap10/sync_delay/Constant: equ=P=C
      link override pol1_in1_tap10/sync_delay/Constant1: equ=P=C
      link override pol1_in1_tap10/sync_delay/Constant2: equ=P=C
      link override pol1_in1_tap10/sync_delay/Constant3: equ=P=C
      link override pol1_in1_tap11/sync_delay/Constant: equ=P=C
      link override pol1_in1_tap11/sync_delay/Constant1: equ=P=C
      link override pol1_in1_tap11/sync_delay/Constant2: equ=P=C
      link override pol1_in1_tap11/sync_delay/Constant3: equ=P=C
      link override pol1_in1_tap12/sync_delay/Constant: equ=P=C
      link override pol1_in1_tap12/sync_delay/Constant1: equ=P=C
      link override pol1_in1_tap12/sync_delay/Constant2: equ=P=C
      link override pol1_in1_tap12/sync_delay/Constant3: equ=P=C
      link override pol1_in1_tap13/sync_delay/Constant: equ=P=C
      link override pol1_in1_tap13/sync_delay/Constant1: equ=P=C
      link override pol1_in1_tap13/sync_delay/Constant2: equ=P=C
      link override pol1_in1_tap13/sync_delay/Constant3: equ=P=C
      link override pol1_in1_tap14/sync_delay/Constant: equ=P=C
      link override pol1_in1_tap14/sync_delay/Constant1: equ=P=C
      link override pol1_in1_tap14/sync_delay/Constant2: equ=P=C
      link override pol1_in1_tap14/sync_delay/Constant3: equ=P=C
      link override pol1_in1_tap15/sync_delay/Constant: equ=P=C
      link override pol1_in1_tap15/sync_delay/Constant1: equ=P=C
      link override pol1_in1_tap15/sync_delay/Constant2: equ=P=C
      link override pol1_in1_tap15/sync_delay/Constant3: equ=P=C
      link override pol1_in1_tap2/sync_delay/Constant: equ=P=C
      link override pol1_in1_tap2/sync_delay/Constant1: equ=P=C
      link override pol1_in1_tap2/sync_delay/Constant2: equ=P=C
      link override pol1_in1_tap2/sync_delay/Constant3: equ=P=C
      link override pol1_in1_tap3/sync_delay/Constant: equ=P=C
      link override pol1_in1_tap3/sync_delay/Constant1: equ=P=C
      link override pol1_in1_tap3/sync_delay/Constant2: equ=P=C
      link override pol1_in1_tap3/sync_delay/Constant3: equ=P=C
      link override pol1_in1_tap4/sync_delay/Constant: equ=P=C
      link override pol1_in1_tap4/sync_delay/Constant1: equ=P=C
      link override pol1_in1_tap4/sync_delay/Constant2: equ=P=C
      link override pol1_in1_tap4/sync_delay/Constant3: equ=P=C
      link override pol1_in1_tap5/sync_delay/Constant: equ=P=C
      link override pol1_in1_tap5/sync_delay/Constant1: equ=P=C
      link override pol1_in1_tap5/sync_delay/Constant2: equ=P=C
      link override pol1_in1_tap5/sync_delay/Constant3: equ=P=C
      link override pol1_in1_tap6/sync_delay/Constant: equ=P=C
      link override pol1_in1_tap6/sync_delay/Constant1: equ=P=C
      link override pol1_in1_tap6/sync_delay/Constant2: equ=P=C
      link override pol1_in1_tap6/sync_delay/Constant3: equ=P=C
      link override pol1_in1_tap7/sync_delay/Constant: equ=P=C
      link override pol1_in1_tap7/sync_delay/Constant1: equ=P=C
      link override pol1_in1_tap7/sync_delay/Constant2: equ=P=C
      link override pol1_in1_tap7/sync_delay/Constant3: equ=P=C
      link override pol1_in1_tap8/sync_delay/Constant: equ=P=C
      link override pol1_in1_tap8/sync_delay/Constant1: equ=P=C
      link override pol1_in1_tap8/sync_delay/Constant2: equ=P=C
      link override pol1_in1_tap8/sync_delay/Constant3: equ=P=C
      link override pol1_in1_tap9/sync_delay/Constant: equ=P=C
      link override pol1_in1_tap9/sync_delay/Constant1: equ=P=C
      link override pol1_in1_tap9/sync_delay/Constant2: equ=P=C
      link override pol1_in1_tap9/sync_delay/Constant3: equ=P=C
      link override pol2_in1_first_tap/sync_delay/Constant: equ=P=C
      link override pol2_in1_first_tap/sync_delay/Constant1: equ=P=C
      link override pol2_in1_first_tap/sync_delay/Constant2: equ=P=C
      link override pol2_in1_first_tap/sync_delay/Constant3: equ=P=C
      link override pol2_in1_tap10/sync_delay/Constant: equ=P=C
      link override pol2_in1_tap10/sync_delay/Constant1: equ=P=C
      link override pol2_in1_tap10/sync_delay/Constant2: equ=P=C
      link override pol2_in1_tap10/sync_delay/Constant3: equ=P=C
      link override pol2_in1_tap11/sync_delay/Constant: equ=P=C
      link override pol2_in1_tap11/sync_delay/Constant1: equ=P=C
      link override pol2_in1_tap11/sync_delay/Constant2: equ=P=C
      link override pol2_in1_tap11/sync_delay/Constant3: equ=P=C
      link override pol2_in1_tap12/sync_delay/Constant: equ=P=C
      link override pol2_in1_tap12/sync_delay/Constant1: equ=P=C
      link override pol2_in1_tap12/sync_delay/Constant2: equ=P=C
      link override pol2_in1_tap12/sync_delay/Constant3: equ=P=C
      link override pol2_in1_tap13/sync_delay/Constant: equ=P=C
      link override pol2_in1_tap13/sync_delay/Constant1: equ=P=C
      link override pol2_in1_tap13/sync_delay/Constant2: equ=P=C
      link override pol2_in1_tap13/sync_delay/Constant3: equ=P=C
      link override pol2_in1_tap14/sync_delay/Constant: equ=P=C
      link override pol2_in1_tap14/sync_delay/Constant1: equ=P=C
      link override pol2_in1_tap14/sync_delay/Constant2: equ=P=C
      link override pol2_in1_tap14/sync_delay/Constant3: equ=P=C
      link override pol2_in1_tap15/sync_delay/Constant: equ=P=C
      link override pol2_in1_tap15/sync_delay/Constant1: equ=P=C
      link override pol2_in1_tap15/sync_delay/Constant2: equ=P=C
      link override pol2_in1_tap15/sync_delay/Constant3: equ=P=C
      link override pol2_in1_tap2/sync_delay/Constant: equ=P=C
      link override pol2_in1_tap2/sync_delay/Constant1: equ=P=C
      link override pol2_in1_tap2/sync_delay/Constant2: equ=P=C
      link override pol2_in1_tap2/sync_delay/Constant3: equ=P=C
      link override pol2_in1_tap3/sync_delay/Constant: equ=P=C
      link override pol2_in1_tap3/sync_delay/Constant1: equ=P=C
      link override pol2_in1_tap3/sync_delay/Constant2: equ=P=C
      link override pol2_in1_tap3/sync_delay/Constant3: equ=P=C
      link override pol2_in1_tap4/sync_delay/Constant: equ=P=C
      link override pol2_in1_tap4/sync_delay/Constant1: equ=P=C
      link override pol2_in1_tap4/sync_delay/Constant2: equ=P=C
      link override pol2_in1_tap4/sync_delay/Constant3: equ=P=C
      link override pol2_in1_tap5/sync_delay/Constant: equ=P=C
      link override pol2_in1_tap5/sync_delay/Constant1: equ=P=C
      link override pol2_in1_tap5/sync_delay/Constant2: equ=P=C
      link override pol2_in1_tap5/sync_delay/Constant3: equ=P=C
      link override pol2_in1_tap6/sync_delay/Constant: equ=P=C
      link override pol2_in1_tap6/sync_delay/Constant1: equ=P=C
      link override pol2_in1_tap6/sync_delay/Constant2: equ=P=C
      link override pol2_in1_tap6/sync_delay/Constant3: equ=P=C
      link override pol2_in1_tap7/sync_delay/Constant: equ=P=C
      link override pol2_in1_tap7/sync_delay/Constant1: equ=P=C
      link override pol2_in1_tap7/sync_delay/Constant2: equ=P=C
      link override pol2_in1_tap7/sync_delay/Constant3: equ=P=C
      link override pol2_in1_tap8/sync_delay/Constant: equ=P=C
      link override pol2_in1_tap8/sync_delay/Constant1: equ=P=C
      link override pol2_in1_tap8/sync_delay/Constant2: equ=P=C
      link override pol2_in1_tap8/sync_delay/Constant3: equ=P=C
      link override pol2_in1_tap9/sync_delay/Constant: equ=P=C
      link override pol2_in1_tap9/sync_delay/Constant1: equ=P=C
      link override pol2_in1_tap9/sync_delay/Constant2: equ=P=C
      link override pol2_in1_tap9/sync_delay/Constant3: equ=P=C
  pol1_sum_sq : xps_library/software register  Tag=xps:sw_reg  io_dir=To Processor  arith_type=Unsigned  bitwidth=32  bin_pt=14  sample_period=1  gw_name=i_r303_med_1_pol1_sum_sq_user_data_in
  pol2_sum_sq : xps_library/software register  Tag=xps:sw_reg  io_dir=To Processor  arith_type=Unsigned  bitwidth=32  bin_pt=14  sample_period=1  gw_name=i_r303_med_1_pol2_sum_sq_user_data_in
  pol3_sum_sq : xps_library/software register  Tag=xps:sw_reg  io_dir=To Processor  arith_type=Unsigned  bitwidth=32  bin_pt=14  sample_period=1  gw_name=i_r303_med_1_pol3_sum_sq_user_data_in
  pol4_sum_sq : xps_library/software register  Tag=xps:sw_reg  io_dir=To Processor  arith_type=Unsigned  bitwidth=32  bin_pt=14  sample_period=1  gw_name=i_r303_med_1_pol4_sum_sq_user_data_in
  posedge1 : adcscope_lib/posedge  Tag=Rising Edge Detector  yummy=on
  posedge6 : Subsystem  Tag=Rising Edge Detector
  pulse_ext1 : Subsystem  mask{pulse_len=2^23}
      mask prompts: pulse_len "Length of Pulse"
      mask init:
      | bits = ceil(log2(pulse_len+1));
  pulse_ext2 : Subsystem  mask{pulse_len=2^23}
      mask prompts: pulse_len "Length of Pulse"
      mask init:
      | bits = ceil(log2(pulse_len+1));
  pulse_ext3 : Subsystem  mask{pulse_len=2^23}
      mask prompts: pulse_len "Length of Pulse"
      mask init:
      | bits = ceil(log2(pulse_len+1));
  pulse_ext4 : Subsystem  mask{pulse_len=2^23}
      mask prompts: pulse_len "Length of Pulse"
      mask init:
      | bits = ceil(log2(pulse_len+1));
  snap_xaui_out : Subsystem  mask(snap64){nsamples=11}
      mask prompts: nsamples "No. of samples(2^?)"
      mask help:
      | The <i>snap</i> block provides a packaged solution to capturing data from
      | the FPGA fabric and making it accessible from the CPU.  The block comes in
      | 2 flavors: <i>snap</i> (which captures to a 32 bit wide Shared BRAM), and
      | <i>snap64</i> (which captures to 2x32 bit wide Shared BRAMs to effect a
      | 64 bit capture).
      mask Help: eval('xlWeb([getenv(''MLIB_ROOT''), ''\casper_library\doc\snap_usage.html''])')
  sram_tvg : Subsystem
  sw_override : xps_library/software register  Tag=xps:sw_reg  io_dir=From Processor  arith_type=Unsigned  bitwidth=32  bin_pt=0  sample_period=1  gw_name=i_r303_med_1_sw_override_user_data_out
  sync_gen : Subsystem
  sync_out : xps_library/gpio  Tag=xps:gpio  io_group=iBOB:sma  io_dir=out  arith_type=Unsigned  bitwidth=1  bin_pt=0  bit_index=1  sample_period=1  use_single_ended=off  use_ddr=off  reg_iob=on  reg_clk_phase=0  termination=None
  wires:
  Pulse Generator/1 -> adc0/3
  Constant1/1 -> adc0/4, adc1/4, adc1/3
  Band-Limited White Noise/1 -> adc0/1, adc0/2, adc1/1, adc1/2
  fft_tvg/1(dout) -> dbuf_ct_sram/1
  dbuf_ct_sram/2 -> sram_tvg/2(sync)
  dbuf_ct_sram/1 -> sram_tvg/1(din)
  pfb_fir/1 -> Delay2/1
  pfb_fir1/1 -> Delay4/1
  sync_gen/1(sync) -> [sync_gen]
  sram_tvg/1(dout) -> one_ant_a_time/1(din)
  sram_tvg/2(sync_out) -> one_ant_a_time/2(sync)
  Constant14/1 -> XAUI1/1(rx_get)
  Constant15/1 -> XAUI1/2(rx_reset)
  XAUI1/5(rx_linkdown) -> neg_edge_ext/1(in)
  adc0/13 -> negedge/1(In)
  adc0/14 -> negedge1/1(In)
  adc0/15 -> negedge2/1(In)
  adc0/16 -> negedge3/1(In)
  adc1/13 -> negedge4/1(In)
  adc1/14 -> negedge5/1(In)
  adc1/15 -> negedge6/1(In)
  adc1/16 -> negedge7/1(In)
  sync_gen/2(mrst) -> [mrst]
  [use_sram_tvg] -> sram_tvg/3(use_tvg)
  [use_fft_tvg] -> fft_tvg/3(use_tvg)
  [arm_rst] -> sync_gen/2(arm)
  decat/1(Out1) -> DDC0_0/1
  decat/2(Out2) -> DDC0_0/2
  decat/3(Out3) -> DDC0_0/3
  decat/4(Out4) -> DDC0_0/4
  adc0/1 -> concat/1(In1)
  adc0/2 -> concat/2(In2)
  adc0/3 -> concat/3(In3)
  adc0/4 -> concat/4(In4)
  concat/1(Out1) -> [ant1_pol1_adc]
  [ant1_pol1_adc] -> decat/1(In1)
  concat4/1(Out1) -> [ant1_pol2_adc]
  adc0/5 -> concat4/1(In1)
  adc0/6 -> concat4/2(In2)
  adc0/7 -> concat4/3(In3)
  adc0/8 -> concat4/4(In4)
  concat5/1(Out1) -> [ant2_pol1_adc]
  concat6/1(Out1) -> [ant2_pol2_adc]
  adc1/1 -> concat5/1(In1)
  adc1/2 -> concat5/2(In2)
  adc1/3 -> concat5/3(In3)
  adc1/4 -> concat5/4(In4)
  adc1/5 -> concat6/1(In1)
  adc1/6 -> concat6/2(In2)
  adc1/7 -> concat6/3(In3)
  adc1/8 -> concat6/4(In4)
  [sync_rst] -> Logical7/2
  [ant1_pol2_adc] -> decat1/1(In1)
  decat1/1(Out1) -> DDC0_1/1
  decat1/2(Out2) -> DDC0_1/2
  decat1/3(Out3) -> DDC0_1/3
  decat1/4(Out4) -> DDC0_1/4
  [ant2_pol1_adc] -> decat2/1(In1)
  [ant2_pol2_adc] -> decat3/1(In1)
  decat2/1(Out1) -> DDC0_2/1
  decat2/2(Out2) -> DDC0_2/2
  decat2/3(Out3) -> DDC0_2/3
  decat2/4(Out4) -> DDC0_2/4
  decat3/1(Out1) -> DDC0_3/1
  decat3/2(Out2) -> DDC0_3/2
  decat3/3(Out3) -> DDC0_3/3
  decat3/4(Out4) -> DDC0_3/4
  [sync_gen] -> DDC0_0/5
  [sync_gen] -> DDC0_1/5
  [sync_gen] -> DDC0_2/5
  [sync_gen] -> DDC0_3/5
  [fft_shift] -> fft/2
  [fft_shift] -> fft1/2
  DDC0_0/1 -> [ant1_pol1_ddc]
  DDC0_0/2 -> [sync_ant1_ddc]
  [sync_ant1_ddc] -> pfb_fir/1
  [ant1_pol1_ddc] -> pfb_fir/2
  [ant1_pol2_ddc] -> pfb_fir/3
  DDC0_1/1 -> [ant1_pol2_ddc]
  DDC0_2/1 -> [ant2_pol1_ddc]
  DDC0_2/2 -> [sync_ant2_ddc]
  DDC0_3/1 -> [ant2_pol2_ddc]
  [sync_ant2_ddc] -> pfb_fir1/1
  [ant2_pol1_ddc] -> pfb_fir1/2
  [ant2_pol2_ddc] -> pfb_fir1/3
  fft/1 -> [sync_ant1_fft]
  fft/2 -> [ant1_pol1_fft]
  fft/3 -> [ant1_pol2_fft]
  fft1/2 -> [ant2_pol1_fft]
  fft1/3 -> [ant2_pol2_fft]
  fft_tvg/2(sync_out) -> dbuf_ct_sram/2
  one_ant_a_time/1(dout) -> [ant12_pol12_reorder]
  one_ant_a_time/2(sync_out) -> [sync_reorder]
  [ant12_pol12_rnd] -> fft_tvg/1(din)
  [sync_rnd] -> fft_tvg/2(sync)
  XAUI1/1(rx_data) -> Slice1/1, Slice2/1
  Register/1 -> [xaui_data]
  calc_adc_sum_sq1/1(sum_sq) -> pol1_sum_sq/1, Slice11/1
  pfb_fir/2 -> downshift/1(din)
  downshift/1(dout) -> fft/3
  pfb_fir/3 -> downshift1/1(din)
  downshift1/1(dout) -> fft/4
  pfb_fir1/2 -> downshift2/1(din)
  downshift2/1(dout) -> fft1/3
  pfb_fir1/3 -> downshift3/1(din)
  downshift3/1(dout) -> fft1/4
  eq_ant1/1(dout) -> [ant1_pol12_rnd]
  eq_ant1/2(sync_out) -> [sync1_rnd]
  [ant1_pol1_fft] -> eq_ant1/1(pol1)
  [ant1_pol2_fft] -> eq_ant1/2(pol2)
  [sync_ant1_fft] -> eq_ant1/3(sync)
  Slice1/1 -> Register/1
  [eq_data_1] -> eq_ant1/4(coeff)
  [eq_en_1] -> eq_ant1/5(coeff_we)
  [eq_addr_1] -> eq_ant1/6(coeff_addr)
  Delay2/1 -> fft/1
  Delay4/1 -> fft1/1
  XAUI1/4(rx_valid) -> Logical/1
  Inverter/1 -> Logical/2
  Logical/1 -> Delay/1, Register/2, Register1/2
  Slice2/1 -> Register1/1
  Register1/1 -> [xaui_addr]
  neg_edge_ext/1(out) -> Inverter/1, [xaui_link_down]
  clk_div_2/1 -> clk_out/1
  Delay/1 -> [xaui_en]
  adc0/9 -> Logical1/1
  adc0/10 -> Logical1/2
  adc0/11 -> Logical1/3
  adc0/12 -> Logical1/4
  adc1/9 -> Logical2/1
  adc1/10 -> Logical2/2
  adc1/11 -> Logical2/3
  adc1/12 -> Logical2/4
  Logical1/1 -> [adc0_clip]
  Logical2/1 -> [adc1_clip]
  [adc0_clip] -> Logical6/1
  [adc1_clip] -> Logical6/2
  sync_gen/3(armed) -> [armed]
  Logical6/1 -> pulse_ext3/1(in)
  pulse_ext3/1(out) -> led5_adc_clip/1
  eq_ant1/3(clip) -> [eq1_clip]
  [ant1_pol1_adc] -> calc_adc_sum_sq1/1(pol_in)
  calc_adc_sum_sq2/1(sum_sq) -> pol2_sum_sq/1, Slice12/1
  calc_adc_sum_sq3/1(sum_sq) -> pol3_sum_sq/1, Slice14/1
  calc_adc_sum_sq4/1(sum_sq) -> pol4_sum_sq/1, Slice15/1
  posedge1/1 -> calc_adc_sum_sq1/2(accum_rst), calc_adc_sum_sq2/2(accum_rst), calc_adc_sum_sq3/2(accum_rst), calc_adc_sum_sq4/2(accum_rst)
  [ant1_pol2_adc] -> calc_adc_sum_sq2/1(pol_in)
  [ant2_pol1_adc] -> calc_adc_sum_sq3/1(pol_in)
  [ant2_pol2_adc] -> calc_adc_sum_sq4/1(pol_in)
  pulse_ext2/1(out) -> led2_sync/1
  [sync_gen] -> pulse_ext2/1(in)
  pulse_ext1/1(out) -> led0_mrst/1
  [mrst] -> pulse_ext1/1(in)
  [armed] -> led1_arm/1
  XAUI1/6(tx_full) -> [xaui_buffer_overflow]
  [xaui_link_down] -> led6_link_dn/1
  pulse_ext4/1(out) -> led4_eq_clip/1
  [eq_clip] -> pulse_ext4/1(in)
  [xaui_buffer_overflow] -> led7_xaui_overlfow/1
  Slice11/1 -> Concat/1
  Slice12/1 -> Concat/2
  Slice14/1 -> Concat/3
  Slice15/1 -> Concat/4
  Concat/1 -> [adc_levels], Slice10/1, Slice13/1
  Counter/1 -> Slice16/1
  Slice16/1 -> posedge1/1
  Logical7/1 -> posedge6/1(In)
  Logical4/1 -> [sync_adc1]
  Logical3/1 -> [sync_adc0]
  [sync_adc0] -> Logical7/1
  [sync_adc1] -> Logical7/3
  [sync_reorder] -> packetiser1/2(sync_in)
  [mrst] -> packetiser1/3(mrst_in)
  packetiser1/1(data_out) -> mux_adc_levels/1(data_in)
  packetiser1/2(valid_out) -> mux_adc_levels/2(valid_in)
  packetiser1/3(header_out) -> mux_adc_levels/3(header)
  packetiser1/4(eof) -> mux_adc_levels/4(eof)
  packetiser1/5(sync_out) -> mux_adc_levels/5(sync)
  mux_adc_levels/1(data_out) -> snap_xaui_out/1(data_in), XAUI1/3(tx_data)
  mux_adc_levels/2(oob) -> Slice4/1, snap_xaui_out/2(oob_in), XAUI1/4(tx_outofband)
  mux_adc_levels/3(valid_out) -> snap_xaui_out/4(we), Logical8/2, XAUI1/5(tx_valid)
  [mrst] -> mux_adc_levels/6(mrst)
  [adc_levels] -> mux_adc_levels/7(adc_power)
  [mrst] -> clk_div_2/1
  [sync_reorder] -> sync_out/1
  Logical8/1 -> snap_xaui_out/3(trig)
  Slice4/1 -> Logical8/1
  Slice10/1 -> adc_lev1/1
  Slice13/1 -> adc_lev2/1
  [ant12_pol12_reorder] -> packetiser1/1(data_in)
  Constant19/1 -> sw_override/1
  sw_override/1 -> Slice5/1, Slice3/1
  Slice5/1 -> Mux7/1, Mux6/1, Mux1/1
  [xaui_addr] -> Mux7/2
  [xaui_data] -> Mux6/2
  data/1 -> Mux6/3
  Constant2/1 -> address/1
  Constant3/1 -> data/1
  address/1 -> Mux7/3
  [xaui_en] -> Mux1/2
  Mux1/1 -> [ctl_en]
  Mux6/1 -> [ctl_data]
  Mux7/1 -> [ctl_addr]
  Slice3/1 -> Mux1/3
  eq_coeff1/1(data_out) -> [eq_data_1]
  eq_coeff1/2(addr_out) -> [eq_addr_1]
  eq_coeff1/3(valid_out) -> [eq_en_1]
  eq_coeff2/1(data_out) -> [eq_data_2]
  eq_coeff2/2(addr_out) -> [eq_addr_2]
  eq_coeff2/3(valid_out) -> [eq_en_2]
  [ctl_data] -> Slice18/1
  [ctl_addr] -> eq_coeff1/2(addr_in)
  [ctl_en] -> eq_coeff1/3(valid_in)
  [ctl_data] -> Slice19/1
  [ctl_addr] -> eq_coeff2/2(addr_in)
  [ctl_en] -> eq_coeff2/3(valid_in)
  Slice9/1 -> [use_sram_tvg]
  Slice8/1 -> [use_fft_tvg]
  Slice7/1 -> [arm_rst]
  Slice6/1 -> [sync_rst]
  Slice21/1 -> [fft_shift]
  Slice17/1 -> [input_sel]
  Delay1/1 -> Slice9/1, Slice8/1, Slice7/1, Slice6/1, Slice21/1, Slice17/1
  Feng_ctl/1(data_out) -> Delay1/1
  [ctl_data] -> Feng_ctl/1(data_in)
  [ctl_addr] -> Feng_ctl/2(addr_in)
  [ctl_en] -> Feng_ctl/3(valid_in)
  eq_ant2/1(dout) -> [ant2_pol12_rnd]
  eq_ant2/2(sync_out) -> [sync2_rnd]
  eq_ant2/3(clip) -> [eq2_clip]
  Logical5/1 -> [eq_clip]
  Concat3/1 -> [ant12_pol12_rnd]
  [ant2_pol1_fft] -> eq_ant2/1(pol1)
  [ant2_pol2_fft] -> eq_ant2/2(pol2)
  [sync_ant2_fft] -> eq_ant2/3(sync)
  [eq_data_2] -> eq_ant2/4(coeff)
  [eq_en_2] -> eq_ant2/5(coeff_we)
  [eq_addr_2] -> eq_ant2/6(coeff_addr)
  fft1/1 -> [sync_ant2_fft]
  [ant1_pol12_rnd] -> Concat3/1
  [ant2_pol12_rnd] -> Concat3/2
  [eq1_clip] -> Logical5/1
  [eq2_clip] -> Logical5/2
  [sync1_rnd] -> [sync_rnd]
  Slice18/1 -> eq_coeff1/1(data_in)
  Slice19/1 -> eq_coeff2/1(data_in)
  negedge4/1(Out) -> Logical4/1
  negedge5/1(Out) -> Logical4/2
  negedge6/1(Out) -> Logical4/3
  negedge7/1(Out) -> Logical4/4
  posedge6/1(Out) -> sync_gen/1(rst)
  negedge/1(Out) -> Logical3/1
  negedge1/1(Out) -> Logical3/2
  negedge2/1(Out) -> Logical3/3
  negedge3/1(Out) -> Logical3/4
